simulink model "Logging_from_phone"  (R2023b)
settings: Solver=ode3  StartTime=0.0  StopTime=60  RelTol=1e-3
libraries: androiduilib x3, androidsensorlib x2, androidaudiovideolib x2
PreSaveFcn:
  | set_param(gcs, 'Location',[35 56 895 605])
settings Model: SimulationMode=external  ExtModeTrigDuration=100  Creator=The MathWorks, Inc.  LastModifiedBy=jay
settings SolverCC: AlgebraicLoopSolver=TrustRegion
settings DataIOCC: LimitDataPoints=on  SaveFormat=StructureWithTime  ReturnWorkspaceOutputs=off  LoggingToFile=on
settings OptimizationCC: LifeSpan=1  MaxStackSize=64
settings DebuggingCC: UnderspecifiedInitializationDetection=Classic  MergeDetectMultiDrivingBlocksExec=none  ParameterPrecisionLossMsg=none  UnconnectedInputMsg=warning  UnconnectedOutputMsg=warning  UnconnectedLineMsg=warning  AllowSymbolicDim=off  SFUnexpectedBacktrackingDiag=warning  SFNoUnconditionalDefaultTransitionDiag=warning  SFExecutionAtInitializationDiag=none  ArithmeticOperatorsInVariantConditions=warning
settings HardwareCC: ProdBitPerPointer=32  ProdLargestAtomicInteger=Long  ProdLargestAtomicFloat=Double  ProdWordSize=32  ProdHWDeviceType=ARM Compatible->ARM Cortex  TargetLargestAtomicInteger=Long  TargetLargestAtomicFloat=Double  TargetEndianess=LittleEndian  TargetHWDeviceType=ARM Compatible->ARM Cortex  UseEmbeddedCoderFeatures=off  UseSimulinkCoderFeatures=off
settings ModelReferenceCC: EnableRefExpFcnMdlSchedulingChecks=on  PropagateSignalLabelsOutOfModel=off
settings SFSimCC: SimUseLocalCustomCode=off  CustomCodeUndefinedFunction=UseInterfaceOnly
settings RTWCC: Description=Embedded Coder  SystemTargetFile=ert.tlc  HardwareBoard=Android Device  TemplateMakefile=ert_default_tmf  GenerateReport=on  RTWVerbose=off  RTWUseLocalCustomCode=off  Toolchain=Android SDK/NDK Tools  LaunchReport=on
settings CodeAppCC: ForceParamTrailComments=on  OperatorAnnotations=on  MangleLength=10  StateflowObjectComments=on  MATLABSourceComments=on
settings ERTTargetCC: MultiwordLength=2048  ERTCustomFileBanners=off  SupportContinuousTime=on  SupportNonInlinedSFcns=on  RemoveResetFunc=off  ModelStepFunctionPrototypeControlCompliant=off
settings ConfigComp: CovMetricSettings=dw  CovSaveCumulativeToWorkspaceVar=on  CovSaveSingleToWorkspaceVar=on  CovExternalEMLEnable=off  CovSFcnEnable=off

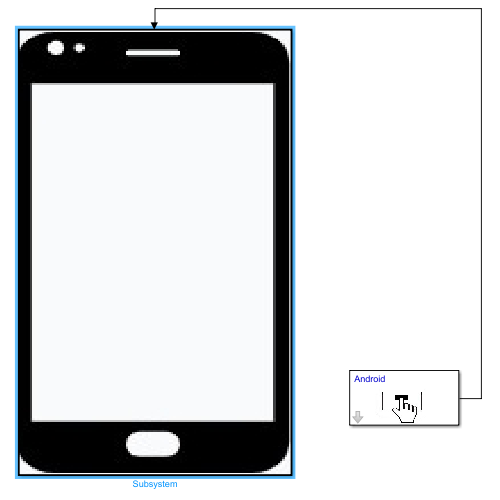
[thumbnail: Simulink's stored preview of the top-level diagram]
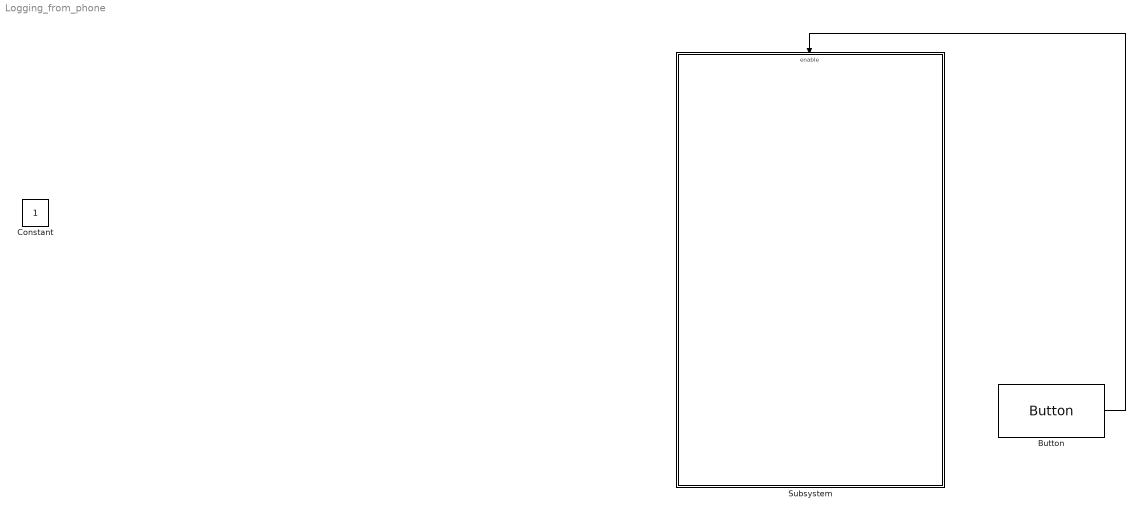
== system Logging_from_phone ==
  Button : androiduilib/Button  ButtonState=Not pressed  ButtonId=Logging_from_phone/Button  State=off  SampleTime=0.1  BlockPlatform=Android
  Subsystem : Subsystem
      mask Display: image('phone.jpg');
  Constant : Constant  IOType=siggen
  wires:
  Button/1 -> Subsystem/Enable

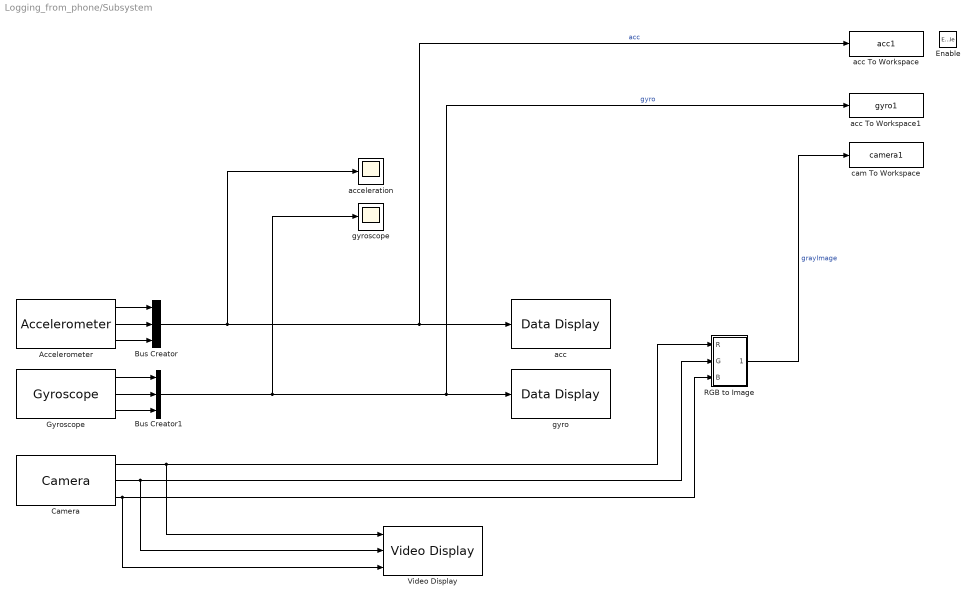
== system Logging_from_phone/Subsystem ==
  Enable : EnablePort
  " cam To Workspace" : ToWorkspace  VariableName=camera1  SaveFormat=Structure With Time  SampleTime=-1
  Accelerometer : androidsensorlib/Accelerometer  OutputVector=off  SampleTime=0.1  BlockPlatform=Android
  Bus Creator : BusCreator  Inputs=3
  Bus Creator1 : BusCreator  Inputs=3
  Camera : androidaudiovideolib/Camera  CameraLocation=Back  CameraResolutions=Back - 640x480  Width=640  Height=480  SampleTime=0.1  BlockPlatform=Android
  Gyroscope : androidsensorlib/Gyroscope  OutputVector=off  SampleTime=0.1  BlockPlatform=Android
  RGB to Image : Subsystem
  Video Display : androidaudiovideolib/Video Display  BlockPlatform=Android
  acc : androiduilib/Data Display  DataDisplayId=Logging_from_phone/Subsystem/acc  Format=Float  Precision=6  SimulateUsing=Code generation  blockPlatform=Android
  acc To Workspace : ToWorkspace  VariableName=acc1  SaveFormat=Structure With Time  SampleTime=-1
  acc To Workspace1 : ToWorkspace  VariableName=gyro1  SaveFormat=Structure With Time  SampleTime=-1
  acceleration : Scope
  gyro : androiduilib/Data Display  DataDisplayId=Logging_from_phone/Subsystem/gyro  Format=Float  Precision=6  SimulateUsing=Code generation  blockPlatform=Android
  gyroscope : Scope
  wires:
  Bus Creator1/1 -> gyroscope/1, acc To Workspace1/1, gyro/1  "gyro"
  Camera/2 -> Video Display/2, RGB to Image/2(G)
  Accelerometer/1 -> Bus Creator/1
  Bus Creator/1 -> acceleration/1, acc To Workspace/1, acc/1  "acc"
  Accelerometer/3 -> Bus Creator/3
  Gyroscope/1 -> Bus Creator1/1
  Camera/1 -> Video Display/1, RGB to Image/1(R)
  Accelerometer/2 -> Bus Creator/2
  Camera/3 -> Video Display/3, RGB to Image/3(B)
  Gyroscope/3 -> Bus Creator1/3
  Gyroscope/2 -> Bus Creator1/2
  RGB to Image/1(Gray) -> " cam To Workspace"/1  "grayImage"

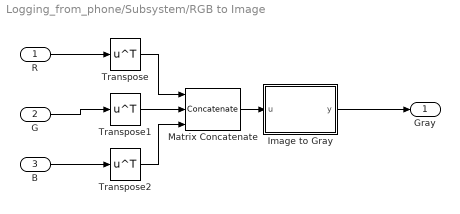
== system Logging_from_phone/Subsystem/RGB to Image ==
  R : Inport
  G : Inport  Port=2
  B : Inport  Port=3
  Image to Gray : MATLAB Function  TreatAsAtomicUnit=on
  Matrix Concatenate : Concatenate  NumInputs=3  Mode=Multidimensional array  ConcatenateDimension=3
  Transpose : Math  Operator=transpose
  Transpose1 : Math  Operator=transpose
  Transpose2 : Math  Operator=transpose
  Gray : Outport
  wires:
  R/1 -> Transpose/1
  Transpose2/1 -> Matrix Concatenate/3
  Matrix Concatenate/1 -> Image to Gray/1(u)
  G/1 -> Transpose1/1
  Transpose/1 -> Matrix Concatenate/1
  Transpose1/1 -> Matrix Concatenate/2
  B/1 -> Transpose2/1
  Image to Gray/1(y) -> Gray/1

== matlab function Logging_from_phone/Subsystem/RGB to Image/Image to Gray ==
  data: u input; y output
function y = fcn(u)

% Insert your algorithm here
y = im2gray(u);
